simulink model "Requirements_Table"  (R2022a)
settings: Solver=FixedStepAuto  StartTime=0.0  StopTime=10.0  FixedStep=1e-3  RelTol=1e-3  EnableMultiTasking=on
settings Model: ExtModeTrigDuration=5  Creator=sabri  LastModifiedBy=Tim
settings SolverCC: AlgebraicLoopSolver=TrustRegion
settings OptimizationCC: EnhancedBackFolding=on  PassReuseOutputArgsAs=Individual arguments  ZeroExternalMemoryAtStartup=off  ZeroInternalMemoryAtStartup=off  MaxStackSize=64  OptimizeBlockOrder=speed  DifferentSizesBufferReuse=on  OptimizationCustomize=off  EfficientTunableParamExpr=on
settings DebuggingCC: ParameterTunabilityLossMsg=error  UnconnectedInputMsg=warning  UnconnectedOutputMsg=warning  UnconnectedLineMsg=warning  SFMachineParentedDataDiag=warning
settings HardwareCC: ProdBitPerPointer=32  ProdBitPerSizeT=32  ProdBitPerPtrDiffT=32  ProdLargestAtomicInteger=Long  ProdLargestAtomicFloat=Double  ProdWordSize=32  ProdHWDeviceType=ARM Compatible->ARM Cortex
settings SFSimCC: MATLABDynamicMemAlloc=off
settings RTWCC: SystemTargetFile=ert.tlc  HardwareBoard=NXP FRDM-K64F  TLCOptions="-aInlineSetEventsForThisBaseRateFcn=TLC_FALSE -aSuppressMultiTaskScheduler=TLC_FALSE  -aRateBasedStepFcn=0"  TemplateMakefile=ert_default_tmf  Toolchain=GNU Tools for ARM Embedded Processors
settings CodeAppCC: ForceParamTrailComments=on  IgnoreCustomStorageClasses=off  OperatorAnnotations=on  SimulinkDataObjDesc=on  SFDataObjDesc=on  InsertBlockDesc=on

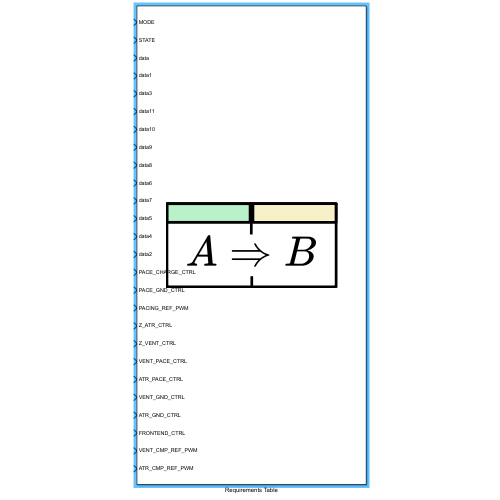
[thumbnail: Simulink's stored preview of the top-level diagram]
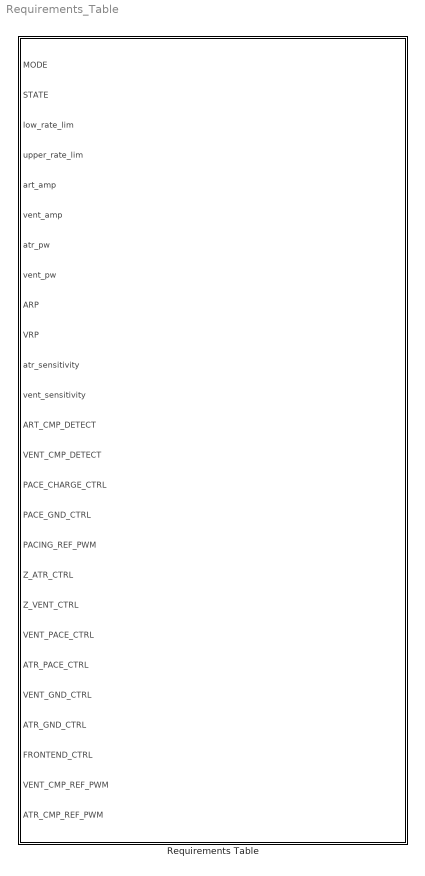
== system Requirements_Table ==
  Requirements Table : Requirements Table  TreatAsAtomicUnit=on

== stateflow chart Requirements_Table/Requirements Table ==
  (default) -> (junction 1073767598)
  (junction 1073767598) -> (junction 1073767599) : {
      | % SF_REQ_REV_07
      | }
  (junction 1073767599) -> (junction 1073767601) : {
      | % HEADER_ASSIGNMENTS
      |
      | }
  (junction 1073767601) -> (junction 1073767603) : {
      | % START_A_4
      | }
  (junction 1073767603) -> (junction 1073767605) : {
      | }
  (junction 1073767605) -> (junction 1073767607)
  (junction 1073767607) -> (junction 1073767609) : {
      | }
  (junction 1073767609) -> (junction 1073767611) : {
      | % END_A_4
      | }
  (junction 1073767611) -> (junction 1073767613) : {
      | % START_R_1
      | }
  (junction 1073767613) -> (junction 1073767615) : {
      | }
  (junction 1073767615) -> (junction 1073767617)
  (junction 1073767617) -> (junction 1073767619) [order 1] : [(((MODE) == (1))) && (((low_rate_lim) >= (30) && (low_rate_lim) <= (175))) && (((upper_rate_lim) >= (50) && (upper_rate_lim) <= (175))) && (((atr_amp) >= (3.5) && (atr_amp) <= (7))) && (((vent_amp) >= (3.5) && (vent_amp) <= (7))) && (((atr_pw) >= (0.1) && (atr_pw) <= (1.9))) && (((vent_pw) >= (0.1) && (vent_pw) <= (1.9))) && (((ARP) >= (150) && (ARP) <= (500))) && (((VRP) >= (150) && (VRP) <= (500))) && (((atr_sensitivity) >= (1) && (atr_sensitivity) <= (10))) && (((vent_sensitivity) >= (1) && (vent_sensitivity) <= (10))) && (((ATR_CMP_DETECT) >= (0) && (ATR_CMP_DETECT) <= (1))) && (((VENT_CMP_DETECT) >= (0) && (VENT_CMP_DETECT) <= (1)))]
  (junction 1073767617) -> (junction 1073767661) [order 2]
  (junction 1073767619) -> (junction 1073767621) : {
      | reqtable_postcondition((((FRONTEND_CTRL) == (0))) && (((VENT_CMP_REF_PWM) == (0))) && (((ATR_CMP_REF_PWM) == (0))), 'R:1');
      |
      |
      | }
  (junction 1073767621) -> (junction 1073767623) : {
      | }
  (junction 1073767623) -> (junction 1073767625) : {
      | % START_R_10
      | }
  (junction 1073767625) -> (junction 1073767627) : {
      | }
  (junction 1073767627) -> (junction 1073767629)
  (junction 1073767629) -> (junction 1073767631) [order 1] : [(((STATE) == (1)))]
  (junction 1073767629) -> (junction 1073767637) [order 2]
  (junction 1073767631) -> (junction 1073767633) : {
      | reqtable_postcondition((((PACE_CHARGE_CTRL) == (0))) && (((PACE_GND_CTRL) == (1))) && (((PACING_REF_PWM) == (vent_amp))) && (((Z_ATR_CTRL) == (0))) && (((Z_VENT_CTRL) == (0))) && (((VENT_PACE_CTRL) == (1))) && (((ATR_PACE_CTRL) == (0))) && (((VENT_GND_CTRL) == (0))) && (((ATR_GND_CTRL) == (0))), 'R:1.1');
      |
      |
      | }
  (junction 1073767633) -> (junction 1073767635) : {
      | }
  (junction 1073767635) -> (junction 1073767637)
  (junction 1073767637) -> (junction 1073767639)
  (junction 1073767639) -> (junction 1073767641) : {
      | % END_R_10
      | }
  (junction 1073767641) -> (junction 1073767643) : {
      | % START_R_16
      | }
  (junction 1073767643) -> (junction 1073767645) : {
      | }
  (junction 1073767645) -> (junction 1073767647)
  (junction 1073767647) -> (junction 1073767649) [order 1] : [(((STATE) == (0)))]
  (junction 1073767647) -> (junction 1073767655) [order 2]
  (junction 1073767649) -> (junction 1073767651) : {
      | reqtable_postcondition((((PACE_CHARGE_CTRL) == (1))) && (((PACE_GND_CTRL) == (1))) && (((PACING_REF_PWM) == (vent_amp))) && (((Z_ATR_CTRL) == (0))) && (((Z_VENT_CTRL) == (0))) && (((VENT_PACE_CTRL) == (0))) && (((ATR_PACE_CTRL) == (0))) && (((VENT_GND_CTRL) == (1))) && (((ATR_GND_CTRL) == (0))), 'R:1.2');
      |
      |
      | }
  (junction 1073767651) -> (junction 1073767653) : {
      | }
  (junction 1073767653) -> (junction 1073767655)
  (junction 1073767655) -> (junction 1073767657)
  (junction 1073767657) -> (junction 1073767659) : {
      | % END_R_16
      | }
  (junction 1073767659) -> (junction 1073767661)
  (junction 1073767661) -> (junction 1073767663)
  (junction 1073767663) -> (junction 1073767665) : {
      | % END_R_1
      | }
  (junction 1073767665) -> (junction 1073767667) : {
      | % START_R_7
      | }
  (junction 1073767667) -> (junction 1073767669) : {
      | }
  (junction 1073767669) -> (junction 1073767671)
  (junction 1073767671) -> (junction 1073767673) [order 1] : [(((MODE) == (2))) && (((low_rate_lim) >= (30) && (low_rate_lim) <= (175))) && (((upper_rate_lim) >= (50) && (upper_rate_lim) <= (175))) && (((atr_amp) >= (3.5) && (atr_amp) <= (7))) && (((vent_amp) >= (3.5) && (vent_amp) <= (7))) && (((atr_pw) >= (0.1) && (atr_pw) <= (1.9))) && (((vent_pw) >= (0.1) && (vent_pw) <= (1.9))) && (((ARP) >= (150) && (ARP) <= (500))) && (((VRP) >= (150) && (VRP) <= (500))) && (((atr_sensitivity) >= (1) && (atr_sensitivity) <= (10))) && (((vent_sensitivity) >= (1) && (vent_sensitivity) <= (10))) && (((ATR_CMP_DETECT) >= (0) && (ATR_CMP_DETECT) <= (1))) && (((VENT_CMP_DETECT) >= (0) && (VENT_CMP_DETECT) <= (1)))]
  (junction 1073767671) -> (junction 1073767715) [order 2]
  (junction 1073767673) -> (junction 1073767675) : {
      | reqtable_postcondition((((FRONTEND_CTRL) == (0))) && (((VENT_CMP_REF_PWM) == (0))) && (((ATR_CMP_REF_PWM) == (0))), 'R:2');
      |
      |
      | }
  (junction 1073767675) -> (junction 1073767677) : {
      | }
  (junction 1073767677) -> (junction 1073767679) : {
      | % START_R_19
      | }
  (junction 1073767679) -> (junction 1073767681) : {
      | }
  (junction 1073767681) -> (junction 1073767683)
  (junction 1073767683) -> (junction 1073767685) [order 1] : [(((STATE) == (1)))]
  (junction 1073767683) -> (junction 1073767691) [order 2]
  (junction 1073767685) -> (junction 1073767687) : {
      | reqtable_postcondition((((PACE_CHARGE_CTRL) == (0))) && (((PACE_GND_CTRL) == (1))) && (((PACING_REF_PWM) == (atr_amp))) && (((Z_ATR_CTRL) == (0))) && (((Z_VENT_CTRL) == (0))) && (((VENT_PACE_CTRL) == (0))) && (((ATR_PACE_CTRL) == (1))) && (((VENT_GND_CTRL) == (0))) && (((ATR_GND_CTRL) == (0))), 'R:2.1');
      |
      |
      | }
  (junction 1073767687) -> (junction 1073767689) : {
      | }
  (junction 1073767689) -> (junction 1073767691)
  (junction 1073767691) -> (junction 1073767693)
  (junction 1073767693) -> (junction 1073767695) : {
      | % END_R_19
      | }
  (junction 1073767695) -> (junction 1073767697) : {
      | % START_R_25
      | }
  (junction 1073767697) -> (junction 1073767699) : {
      | }
  (junction 1073767699) -> (junction 1073767701)
  (junction 1073767701) -> (junction 1073767703) [order 1] : [(((STATE) == (0)))]
  (junction 1073767701) -> (junction 1073767709) [order 2]
  (junction 1073767703) -> (junction 1073767705) : {
      | reqtable_postcondition((((PACE_CHARGE_CTRL) == (1))) && (((PACE_GND_CTRL) == (1))) && (((PACING_REF_PWM) == (atr_amp))) && (((Z_ATR_CTRL) == (0))) && (((Z_VENT_CTRL) == (0))) && (((VENT_PACE_CTRL) == (0))) && (((ATR_PACE_CTRL) == (0))) && (((VENT_GND_CTRL) == (0))) && (((ATR_GND_CTRL) == (1))), 'R:2.2');
      |
      |
      | }
  (junction 1073767705) -> (junction 1073767707) : {
      | }
  (junction 1073767707) -> (junction 1073767709)
  (junction 1073767709) -> (junction 1073767711)
  (junction 1073767711) -> (junction 1073767713) : {
      | % END_R_25
      | }
  (junction 1073767713) -> (junction 1073767715)
  (junction 1073767715) -> (junction 1073767717)
  (junction 1073767717) -> (junction 1073767719) : {
      | % END_R_7
      | }
  (junction 1073767719) -> (junction 1073767721) : {
      | % START_R_28
      | }
  (junction 1073767721) -> (junction 1073767723) : {
      | }
  (junction 1073767723) -> (junction 1073767725)
  (junction 1073767725) -> (junction 1073767727) [order 1] : [(((MODE) == (3))) && (((low_rate_lim) >= (30) && (low_rate_lim) <= (175))) && (((upper_rate_lim) >= (50) && (upper_rate_lim) <= (175))) && (((atr_amp) >= (3.5) && (atr_amp) <= (7))) && (((vent_amp) >= (3.5) && (vent_amp) <= (7))) && (((atr_pw) >= (0.1) && (atr_pw) <= (1.9))) && (((vent_pw) >= (0.1) && (vent_pw) <= (1.9))) && (((ARP) >= (150) && (ARP) <= (500))) && (((VRP) >= (150) && (VRP) <= (500))) && (((atr_sensitivity) >= (1) && (atr_sensitivity) <= (10))) && (((vent_sensitivity) >= (1) && (vent_sensitivity) <= (10))) && (((ATR_CMP_DETECT) >= (0) && (ATR_CMP_DETECT) <= (1))) && (((VENT_CMP_DETECT) >= (0) && (VENT_CMP_DETECT) <= (1)))]
  (junction 1073767725) -> (junction 1073767787) [order 2]
  (junction 1073767727) -> (junction 1073767729) : {
      | reqtable_postcondition((((ATR_CMP_REF_PWM) == (0))), 'R:3');
      |
      |
      | }
  (junction 1073767729) -> (junction 1073767731) : {
      | }
  (junction 1073767731) -> (junction 1073767733) : {
      | % START_R_34
      | }
  (junction 1073767733) -> (junction 1073767735) : {
      | }
  (junction 1073767735) -> (junction 1073767737)
  (junction 1073767737) -> (junction 1073767739) [order 1] : [(((STATE) == (1)))]
  (junction 1073767737) -> (junction 1073767745) [order 2]
  (junction 1073767739) -> (junction 1073767741) : {
      | reqtable_postcondition((((PACE_CHARGE_CTRL) == (0))) && (((PACE_GND_CTRL) == (1))) && (((PACING_REF_PWM) == (vent_amp))) && (((Z_ATR_CTRL) == (0))) && (((Z_VENT_CTRL) == (0))) && (((VENT_PACE_CTRL) == (1))) && (((ATR_PACE_CTRL) == (0))) && (((VENT_GND_CTRL) == (0))) && (((ATR_GND_CTRL) == (0))) && (((FRONTEND_CTRL) == (1))) && (((VENT_CMP_REF_PWM) == (vent_sensitivity))), 'R:3.1');
      |
      |
      | }
  (junction 1073767741) -> (junction 1073767743) : {
      | }
  (junction 1073767743) -> (junction 1073767745)
  (junction 1073767745) -> (junction 1073767747)
  (junction 1073767747) -> (junction 1073767749) : {
      | % END_R_34
      | }
  (junction 1073767749) -> (junction 1073767751) : {
      | % START_R_37
      | }
  (junction 1073767751) -> (junction 1073767753) : {
      | }
  (junction 1073767753) -> (junction 1073767755)
  (junction 1073767755) -> (junction 1073767757) [order 1] : [(((STATE) == (0)))]
  (junction 1073767755) -> (junction 1073767763) [order 2]
  (junction 1073767757) -> (junction 1073767759) : {
      | reqtable_postcondition((((PACE_CHARGE_CTRL) == (1))) && (((PACE_GND_CTRL) == (1))) && (((PACING_REF_PWM) == (vent_amp))) && (((Z_ATR_CTRL) == (0))) && (((Z_VENT_CTRL) == (0))) && (((VENT_PACE_CTRL) == (0))) && (((ATR_PACE_CTRL) == (0))) && (((VENT_GND_CTRL) == (1))) && (((ATR_GND_CTRL) == (0))) && (((FRONTEND_CTRL) == (1))) && (((VENT_CMP_REF_PWM) == (vent_sensitivity))), 'R:3.2');
      |
      |
      | }
  (junction 1073767759) -> (junction 1073767761) : {
      | }
  (junction 1073767761) -> (junction 1073767763)
  (junction 1073767763) -> (junction 1073767765)
  (junction 1073767765) -> (junction 1073767767) : {
      | % END_R_37
      | }
  (junction 1073767767) -> (junction 1073767769) : {
      | % START_R_40
      | }
  (junction 1073767769) -> (junction 1073767771) : {
      | }
  (junction 1073767771) -> (junction 1073767773)
  (junction 1073767773) -> (junction 1073767775) [order 1] : [(((STATE) == (2)))]
  (junction 1073767773) -> (junction 1073767781) [order 2]
  (junction 1073767775) -> (junction 1073767777) : {
      | reqtable_postcondition((((PACE_CHARGE_CTRL) == (1))) && (((PACE_GND_CTRL) == (1))) && (((PACING_REF_PWM) == (vent_amp))) && (((Z_ATR_CTRL) == (0))) && (((Z_VENT_CTRL) == (0))) && (((VENT_PACE_CTRL) == (0))) && (((ATR_PACE_CTRL) == (0))) && (((VENT_GND_CTRL) == (1))) && (((ATR_GND_CTRL) == (0))) && (((FRONTEND_CTRL) == (0))) && (((VENT_CMP_REF_PWM) == (vent_sensitivity))), 'R:3.3');
      |
      |
      | }
  (junction 1073767777) -> (junction 1073767779) : {
      | }
  (junction 1073767779) -> (junction 1073767781)
  (junction 1073767781) -> (junction 1073767783)
  (junction 1073767783) -> (junction 1073767785) : {
      | % END_R_40
      | }
  (junction 1073767785) -> (junction 1073767787)
  (junction 1073767787) -> (junction 1073767789)
  (junction 1073767789) -> (junction 1073767791) : {
      | % END_R_28
      | }
  (junction 1073767791) -> (junction 1073767793) : {
      | % START_R_31
      | }
  (junction 1073767793) -> (junction 1073767795) : {
      | }
  (junction 1073767795) -> (junction 1073767797)
  (junction 1073767797) -> (junction 1073767799) [order 1] : [(((MODE) == (4))) && (((low_rate_lim) >= (30) && (low_rate_lim) <= (175))) && (((upper_rate_lim) >= (50) && (upper_rate_lim) <= (175))) && (((atr_amp) >= (3.5) && (atr_amp) <= (7))) && (((vent_amp) >= (3.5) && (vent_amp) <= (7))) && (((atr_pw) >= (0.1) && (atr_pw) <= (1.9))) && (((vent_pw) >= (0.1) && (vent_pw) <= (1.9))) && (((ARP) >= (150) && (ARP) <= (500))) && (((VRP) >= (150) && (VRP) <= (500))) && (((atr_sensitivity) >= (1) && (atr_sensitivity) <= (10))) && (((vent_sensitivity) >= (1) && (vent_sensitivity) <= (10))) && (((ATR_CMP_DETECT) >= (0) && (ATR_CMP_DETECT) <= (1))) && (((VENT_CMP_DETECT) >= (0) && (VENT_CMP_DETECT) <= (1)))]
  (junction 1073767797) -> (junction 1073767859) [order 2]
  (junction 1073767799) -> (junction 1073767801) : {
      | reqtable_postcondition((((VENT_CMP_REF_PWM) == (0))), 'R:4');
      |
      |
      | }
  (junction 1073767801) -> (junction 1073767803) : {
      | }
  (junction 1073767803) -> (junction 1073767805) : {
      | % START_R_52
      | }
  (junction 1073767805) -> (junction 1073767807) : {
      | }
  (junction 1073767807) -> (junction 1073767809)
  (junction 1073767809) -> (junction 1073767811) [order 1] : [(((STATE) == (1)))]
  (junction 1073767809) -> (junction 1073767817) [order 2]
  (junction 1073767811) -> (junction 1073767813) : {
      | reqtable_postcondition((((PACE_CHARGE_CTRL) == (0))) && (((PACE_GND_CTRL) == (1))) && (((PACING_REF_PWM) == (atr_amp))) && (((Z_ATR_CTRL) == (0))) && (((Z_VENT_CTRL) == (0))) && (((VENT_PACE_CTRL) == (0))) && (((ATR_PACE_CTRL) == (1))) && (((VENT_GND_CTRL) == (0))) && (((ATR_GND_CTRL) == (0))) && (((FRONTEND_CTRL) == (1))) && (((ATR_CMP_REF_PWM) == (atr_sensitivity))), 'R:4.1');
      |
      |
      | }
  (junction 1073767813) -> (junction 1073767815) : {
      | }
  (junction 1073767815) -> (junction 1073767817)
  (junction 1073767817) -> (junction 1073767819)
  (junction 1073767819) -> (junction 1073767821) : {
      | % END_R_52
      | }
  (junction 1073767821) -> (junction 1073767823) : {
      | % START_R_55
      | }
  (junction 1073767823) -> (junction 1073767825) : {
      | }
  (junction 1073767825) -> (junction 1073767827)
  (junction 1073767827) -> (junction 1073767829) [order 1] : [(((STATE) == (0)))]
  (junction 1073767827) -> (junction 1073767835) [order 2]
  (junction 1073767829) -> (junction 1073767831) : {
      | reqtable_postcondition((((PACE_CHARGE_CTRL) == (1))) && (((PACE_GND_CTRL) == (1))) && (((PACING_REF_PWM) == (atr_amp))) && (((Z_ATR_CTRL) == (0))) && (((Z_VENT_CTRL) == (0))) && (((VENT_PACE_CTRL) == (0))) && (((ATR_PACE_CTRL) == (0))) && (((VENT_GND_CTRL) == (0))) && (((ATR_GND_CTRL) == (1))) && (((FRONTEND_CTRL) == (1))) && (((ATR_CMP_REF_PWM) == (atr_sensitivity))), 'R:4.2');
      |
      |
      | }
  (junction 1073767831) -> (junction 1073767833) : {
      | }
  (junction 1073767833) -> (junction 1073767835)
  (junction 1073767835) -> (junction 1073767837)
  (junction 1073767837) -> (junction 1073767839) : {
      | % END_R_55
      | }
  (junction 1073767839) -> (junction 1073767841) : {
      | % START_R_58
      | }
  (junction 1073767841) -> (junction 1073767843) : {
      | }
  (junction 1073767843) -> (junction 1073767845)
  (junction 1073767845) -> (junction 1073767847) [order 1] : [(((STATE) == (2)))]
  (junction 1073767845) -> (junction 1073767853) [order 2]
  (junction 1073767847) -> (junction 1073767849) : {
      | reqtable_postcondition((((PACE_CHARGE_CTRL) == (1))) && (((PACE_GND_CTRL) == (1))) && (((PACING_REF_PWM) == (atr_amp))) && (((Z_ATR_CTRL) == (0))) && (((Z_VENT_CTRL) == (0))) && (((VENT_PACE_CTRL) == (0))) && (((ATR_PACE_CTRL) == (0))) && (((VENT_GND_CTRL) == (0))) && (((ATR_GND_CTRL) == (1))) && (((FRONTEND_CTRL) == (0))) && (((ATR_CMP_REF_PWM) == (atr_sensitivity))), 'R:4.3');
      |
      |
      | }
  (junction 1073767849) -> (junction 1073767851) : {
      | }
  (junction 1073767851) -> (junction 1073767853)
  (junction 1073767853) -> (junction 1073767855)
  (junction 1073767855) -> (junction 1073767857) : {
      | % END_R_58
      | }
  (junction 1073767857) -> (junction 1073767859)
  (junction 1073767859) -> (junction 1073767861)
  (junction 1073767861) -> (junction 1073767863) : {
      | % END_R_31
      | }
  data: MODE input; STATE input; low_rate_lim input; upper_rate_lim input; art_amp input; vent_amp input; atr_pw input; vent_pw input; ARP input; VRP input; atr_sensitivity input; vent_sensitivity input; ART_CMP_DETECT input; VENT_CMP_DETECT input; PACE_CHARGE_CTRL input; PACE_GND_CTRL input; PACING_REF_PWM input; Z_ATR_CTRL input; Z_VENT_CTRL input; VENT_PACE_CTRL input; ATR_PACE_CTRL input; VENT_GND_CTRL input; ATR_GND_CTRL input; FRONTEND_CTRL input; VENT_CMP_REF_PWM input; ATR_CMP_REF_PWM input
